simulink model "TwoNeuronTest"  (R2016b)
settings: Solver=VariableStepAuto  StartTime=0.0  StopTime=15  RelTol=1e-3  EnableMultiTasking=on
libraries: simulink x2, powerlib_meascontrol x1
settings Model: Creator=ramin  LastModifiedBy=ramin
settings DataIOCC: LimitDataPoints=on
settings OptimizationCC: LifeSpan=inf
settings DebuggingCC: AllowSymbolicDim=off  SFUnexpectedBacktrackingDiag=warning  SFNoUnconditionalDefaultTransitionDiag=warning  SFExecutionAtInitializationDiag=none
settings ModelReferenceCC: PropagateSignalLabelsOutOfModel=off
settings GRTTargetCC: TargetLangStandard=C89/C90 (ANSI)
settings ConfigComp: CovMetricSettings=dw  CovHtmlReporting=on  CovSaveCumulativeToWorkspaceVar=on  CovSaveSingleToWorkspaceVar=on  CovExternalEMLEnable=off

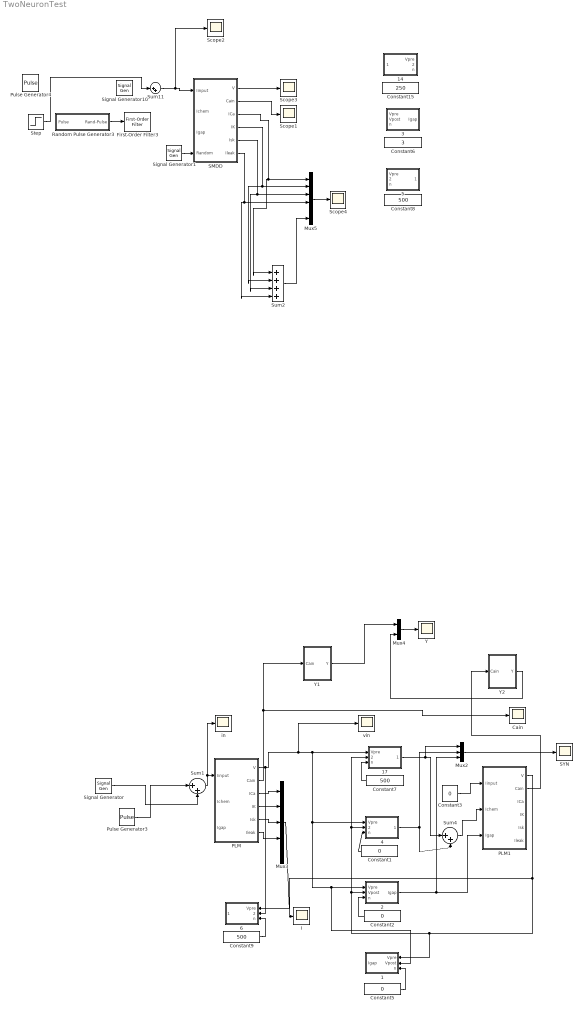
== system TwoNeuronTest ==
  1 : Subsystem
  14 : Subsystem
  17 : Subsystem
  2 : Subsystem
  3 : Subsystem
  4 : Subsystem
  5 : Subsystem
  6 : Subsystem
  Cain : Scope
  Constant{1..3,5} (4 alike) : Constant  Value=0
  Constant15 : Constant  Value=250
  Constant6 : Constant  Value=3
  Constant7 : Constant  Value=500
  Constant8 : Constant  Value=500
  Constant9 : Constant  Value=500
  First-Order Filter3 : powerlib_meascontrol/Filters/First-Order Filter  FilterType=Lowpass  Tc=1  Ts=0  Initialize=off  Vac_Init=[0, 0, 60]  Vdc_Init=0  PlotResponse=off  FreqRange="[0,  200,  1]"
  I : Scope
  Mux2 : Mux  Inputs=3
  Mux3 : Mux  Inputs=5
  Mux4 : Mux  Inputs=2
  Mux5 : Mux  Inputs=6
  PLM : Subsystem
  PLM1 : Subsystem
  Pulse Generator3 : DiscretePulseGenerator  PulseType=Time based  Amplitude=2500  Period=20  PulseWidth=50  PhaseDelay=2
  Pulse Generator4 : DiscretePulseGenerator  PulseType=Time based  Amplitude=2000  Period=200  PulseWidth=80  PhaseDelay=2
  Random Pulse Generator3 : Subsystem
  SMDD : Subsystem
  SYN : Scope
  Scope{1..4} (4 alike) : Scope
  Signal Generator : SignalGenerator  WaveForm=random  Amplitude=0  Frequency=1000000
  Signal Generator1 : SignalGenerator  WaveForm=random  Amplitude=0.5
  Signal Generator10 : SignalGenerator  WaveForm=random  Amplitude=0  Frequency=100
  Step : Step  Time=50  After=2000  SampleTime=0
  Sum1 : Sum  Inputs=|++
  Sum11 : Sum  Inputs=|++
  Sum2 : Sum  Inputs=|++++
  Sum4 : Sum  Inputs=|++
  Y : Scope
  Y1 : Subsystem
  Y2 : Subsystem
  in : Scope
  vin : Scope
  wires:
  PLM/2("Cain ") -> Cain/1, Y1/1(Cain)
  Sum4/1 -> PLM1/2(Ichem)
  Constant1/1 -> 4/3(n)
  Constant7/1 -> 17/3(n)
  Constant2/1 -> 2/3(n)
  4/1(Ichem) -> Sum4/2, Mux2/2
  PLM1/1(V) -> 6/1(Vpre), 1/1(Vpre), 17/2(Vpost), 4/2(Vpost), 2/2(Vpost)
  17/1(Ichem) -> Mux2/1, Sum4/1
  Constant3/1 -> PLM1/1(Iinput)
  PLM1/2("Cain ") -> Y2/1(Cain)
  PLM/1(V) -> vin/1, 17/1(Vpre), 4/1(Vpre), 1/2(Vpost), 2/1(Vpre), 6/2(Vpost)
  2/1(Igap) -> PLM1/3(Igap), Mux2/3
  Mux2/1 -> SYN/1
  Mux3/1 -> I/1
  PLM/3(ICa) -> Mux3/1
  PLM/4(IK) -> Mux3/2
  PLM/5(Isk) -> Mux3/3
  PLM/6(Ileak) -> Mux3/4
  Constant5/1 -> 1/3(n)
  Sum1/1 -> in/1, PLM/1(Iinput)
  Pulse Generator3/1 -> Sum1/1
  Signal Generator/1 -> Sum1/2
  Y1/1(Y) -> Mux4/1
  Mux4/1 -> Y/1
  Y2/1(Y) -> Mux4/2
  Signal Generator1/1 -> SMDD/4(Random)
  Random Pulse Generator3/1(Rand-Pulse) -> First-Order Filter3/1
  Sum11/1 -> Scope2/1, SMDD/1(Iinput)
  Step/1 -> Sum11/1
  SMDD/1(V) -> Scope3/1
  SMDD/2("Cain ") -> Scope1/1
  SMDD/3(ICa) -> Sum2/1, Mux5/1
  SMDD/4(IK) -> Sum2/2, Mux5/2
  SMDD/5(Isk) -> Sum2/3, Mux5/3
  SMDD/6(Ileak) -> Sum2/4, Mux5/4
  Sum2/1 -> Mux5/6
  Mux5/1 -> Scope4/1
  Constant9/1 -> 6/3(n)

== system TwoNeuronTest/1 ==
  Vpre : Inport
  Vpost : Inport  Port=2
  n : Inport  Port=3
  Ggap : Constant  Value=1.02
  Product2 : Product  Inputs=3
  Sum6 : Sum  Inputs=|+-
  Igap : Outport
  wires:
  Vpre/1 -> Sum6/1
  n/1 -> Product2/2
  Sum6/1 -> Product2/1
  Product2/1 -> Igap/1  "Igap"
  Vpost/1 -> Sum6/2
  Ggap/1 -> Product2/3

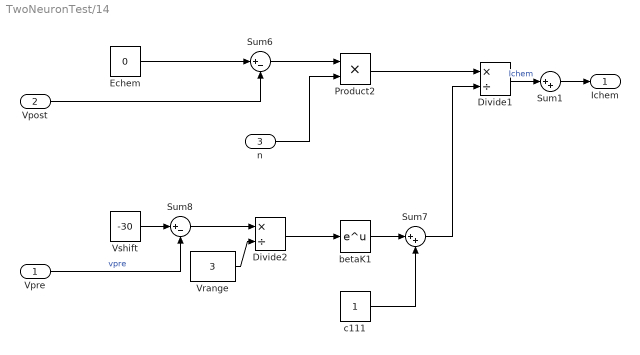
== system TwoNeuronTest/14 ==
  Vpre : Inport
  Vpost : Inport  Port=2
  n : Inport  Port=3
  Divide1 : Product  Inputs=*/
  Divide2 : Product  Inputs=*/
  Echem : Constant  Value=0
  Product2 : Product
  Sum1 : Sum  Inputs=|++
  Sum6 : Sum  Inputs=|+-
  Sum7 : Sum  Inputs=|++
  Sum8 : Sum  Inputs=|+-
  Vrange : Constant  Value=3
  Vshift : Constant  Value=-30
  betaK1 : Math  SaturateOnIntegerOverflow=on
  c111 : Constant
  Ichem : Outport
  wires:
  Echem/1 -> Sum6/1
  n/1 -> Product2/2
  Sum6/1 -> Product2/1
  Product2/1 -> Divide1/1
  betaK1/1 -> Sum7/1
  c111/1 -> Sum7/2
  Vshift/1 -> Sum8/1
  Vpre/1 -> Sum8/2  "vpre"
  Sum8/1 -> Divide2/1
  Vrange/1 -> Divide2/2
  Divide2/1 -> betaK1/1
  Sum7/1 -> Divide1/2
  Divide1/1 -> Sum1/1  "Ichem"
  Vpost/1 -> Sum6/2
  Sum1/1 -> Ichem/1

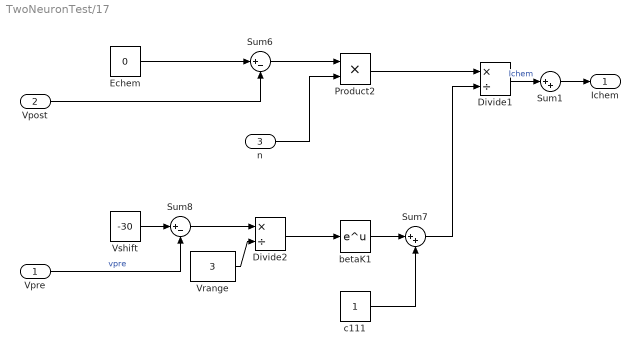
== system TwoNeuronTest/17 ==
  Vpre : Inport
  Vpost : Inport  Port=2
  n : Inport  Port=3
  Divide1 : Product  Inputs=*/
  Divide2 : Product  Inputs=*/
  Echem : Constant  Value=0
  Product2 : Product
  Sum1 : Sum  Inputs=|++
  Sum6 : Sum  Inputs=|+-
  Sum7 : Sum  Inputs=|++
  Sum8 : Sum  Inputs=|+-
  Vrange : Constant  Value=3
  Vshift : Constant  Value=-30
  betaK1 : Math  SaturateOnIntegerOverflow=on
  c111 : Constant
  Ichem : Outport
  wires:
  Echem/1 -> Sum6/1
  n/1 -> Product2/2
  Sum6/1 -> Product2/1
  Product2/1 -> Divide1/1
  betaK1/1 -> Sum7/1
  c111/1 -> Sum7/2
  Vshift/1 -> Sum8/1
  Vpre/1 -> Sum8/2  "vpre"
  Sum8/1 -> Divide2/1
  Vrange/1 -> Divide2/2
  Divide2/1 -> betaK1/1
  Sum7/1 -> Divide1/2
  Divide1/1 -> Sum1/1  "Ichem"
  Vpost/1 -> Sum6/2
  Sum1/1 -> Ichem/1

== system TwoNeuronTest/2 ==
  Vpre : Inport
  Vpost : Inport  Port=2
  n : Inport  Port=3
  Ggap : Constant  Value=1.02
  Product2 : Product  Inputs=3
  Sum6 : Sum  Inputs=|+-
  Igap : Outport
  wires:
  Vpre/1 -> Sum6/1
  n/1 -> Product2/2
  Sum6/1 -> Product2/1
  Product2/1 -> Igap/1  "Igap"
  Vpost/1 -> Sum6/2
  Ggap/1 -> Product2/3

== system TwoNeuronTest/3 ==
  Vpre : Inport
  Vpost : Inport  Port=2
  n : Inport  Port=3
  Ggap : Constant  Value=10
  Product2 : Product  Inputs=3
  Sum6 : Sum  Inputs=|+-
  Igap : Outport
  wires:
  Vpre/1 -> Sum6/1
  n/1 -> Product2/2
  Sum6/1 -> Product2/1
  Product2/1 -> Igap/1  "Igap"
  Vpost/1 -> Sum6/2
  Ggap/1 -> Product2/3

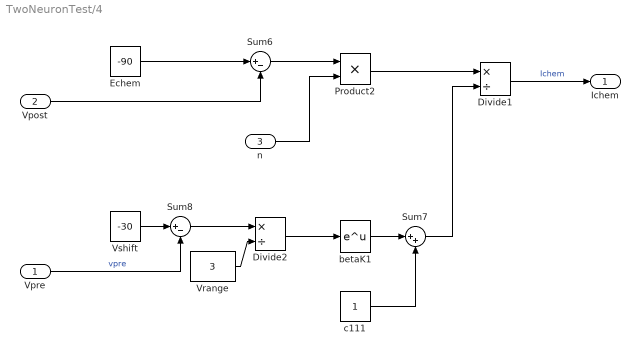
== system TwoNeuronTest/4 ==
  Vpre : Inport
  Vpost : Inport  Port=2
  n : Inport  Port=3
  Divide1 : Product  Inputs=*/
  Divide2 : Product  Inputs=*/
  Echem : Constant  Value=-90
  Product2 : Product
  Sum6 : Sum  Inputs=|+-
  Sum7 : Sum  Inputs=|++
  Sum8 : Sum  Inputs=|+-
  Vrange : Constant  Value=3
  Vshift : Constant  Value=-30
  betaK1 : Math  SaturateOnIntegerOverflow=on
  c111 : Constant
  Ichem : Outport
  wires:
  Echem/1 -> Sum6/1
  n/1 -> Product2/2
  Sum6/1 -> Product2/1
  Product2/1 -> Divide1/1
  betaK1/1 -> Sum7/1
  c111/1 -> Sum7/2
  Vshift/1 -> Sum8/1
  Vpre/1 -> Sum8/2  "vpre"
  Sum8/1 -> Divide2/1
  Vrange/1 -> Divide2/2
  Divide2/1 -> betaK1/1
  Sum7/1 -> Divide1/2
  Divide1/1 -> Ichem/1  "Ichem"
  Vpost/1 -> Sum6/2

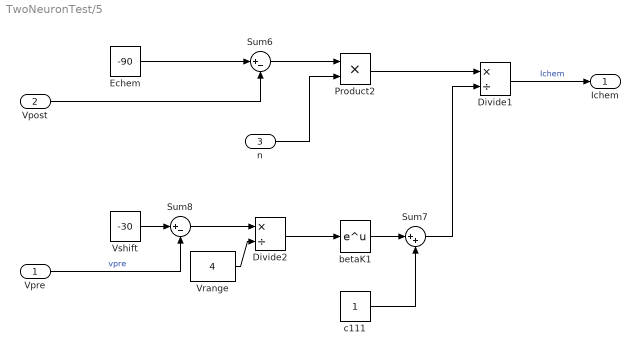
== system TwoNeuronTest/5 ==
  Vpre : Inport
  Vpost : Inport  Port=2
  n : Inport  Port=3
  Divide1 : Product  Inputs=*/
  Divide2 : Product  Inputs=*/
  Echem : Constant  Value=-90
  Product2 : Product
  Sum6 : Sum  Inputs=|+-
  Sum7 : Sum  Inputs=|++
  Sum8 : Sum  Inputs=|+-
  Vrange : Constant  Value=4
  Vshift : Constant  Value=-30
  betaK1 : Math  SaturateOnIntegerOverflow=on
  c111 : Constant
  Ichem : Outport
  wires:
  Echem/1 -> Sum6/1
  n/1 -> Product2/2
  Sum6/1 -> Product2/1
  Product2/1 -> Divide1/1
  betaK1/1 -> Sum7/1
  c111/1 -> Sum7/2
  Vshift/1 -> Sum8/1
  Vpre/1 -> Sum8/2  "vpre"
  Sum8/1 -> Divide2/1
  Vrange/1 -> Divide2/2
  Divide2/1 -> betaK1/1
  Sum7/1 -> Divide1/2
  Divide1/1 -> Ichem/1  "Ichem"
  Vpost/1 -> Sum6/2

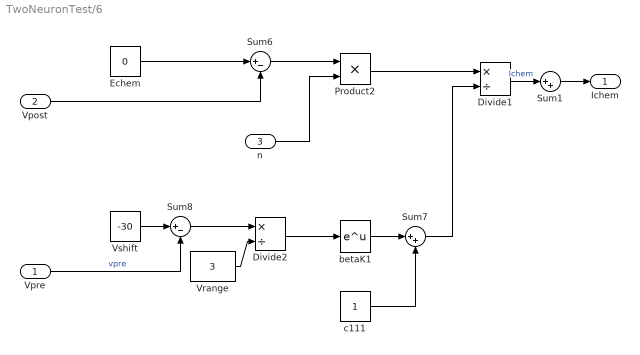
== system TwoNeuronTest/6 ==
  Vpre : Inport
  Vpost : Inport  Port=2
  n : Inport  Port=3
  Divide1 : Product  Inputs=*/
  Divide2 : Product  Inputs=*/
  Echem : Constant  Value=0
  Product2 : Product
  Sum1 : Sum  Inputs=|++
  Sum6 : Sum  Inputs=|+-
  Sum7 : Sum  Inputs=|++
  Sum8 : Sum  Inputs=|+-
  Vrange : Constant  Value=3
  Vshift : Constant  Value=-30
  betaK1 : Math  SaturateOnIntegerOverflow=on
  c111 : Constant
  Ichem : Outport
  wires:
  Echem/1 -> Sum6/1
  n/1 -> Product2/2
  Sum6/1 -> Product2/1
  Product2/1 -> Divide1/1
  betaK1/1 -> Sum7/1
  c111/1 -> Sum7/2
  Vshift/1 -> Sum8/1
  Vpre/1 -> Sum8/2  "vpre"
  Sum8/1 -> Divide2/1
  Vrange/1 -> Divide2/2
  Divide2/1 -> betaK1/1
  Sum7/1 -> Divide1/2
  Divide1/1 -> Sum1/1  "Ichem"
  Vpost/1 -> Sum6/2
  Sum1/1 -> Ichem/1

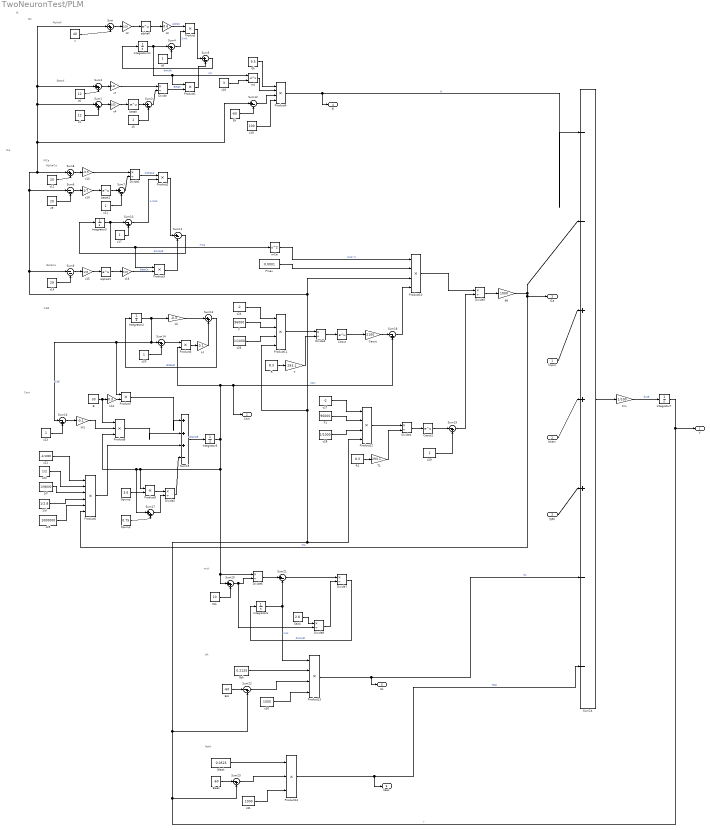
== system TwoNeuronTest/PLM ==
  note: Isk
  note: msk
  note: ICa
  note: Cain
  note: CaB
  note: BetaCa
  note: AlphaCa
  note: MCa
  note: IK
  note: Mk
  note: BetaK
  note: AlphaK
  note: Ileak
  Iinput : Inport
  Ichem : Inport  Port=2
  Igap : Inport  Port=3
  1/F : Constant  Value=1/96000
  1/d : Constant  Value=1/2.8
  B : Constant  Value=30
  Caout : Math  SaturateOnIntegerOverflow=on
  "Caout " : Gain  Gain=2100
  Caout1 : Math  SaturateOnIntegerOverflow=on
  "Cm " : Gain  Gain=1/100
  Divide{,1..8} (9 alike) : Product  Inputs=*/
  "Ek " : Constant  Value=-60
  Eleak : Constant  Value=-60
  Esk : Constant  Value=-60
  F : Constant  Value=96000
  F1 : Constant  Value=96000
  "Gk " : Constant  Value=9.5
  Gleak : Constant  Value=0.0525
  Gpump : Constant  Value=3.6
  Gsk : Constant  Value=0.2125
  Integrator3 : Integrator  InitialCondition=0.001
  Integrator4 : Integrator
  Integrator5 : Integrator
  Integrator6 : Integrator  InitialCondition=1
  Integrator7 : Integrator  InitialCondition=-60
  Integratormk : Integrator
  Kpump : Constant  Value=0.75
  Ksk : Constant  Value=10
  Pmax : Constant  Value=0.0001
  Product{,1..3,5,7,9} (7 alike) : Product
  Product{4,10..13} (5 alike) : Product  Inputs=4
  Product14 : Product  Inputs=3
  Product6 : Product  Inputs=6
  Product8 : Product  Inputs=3
  R : Constant  Value=8.3
  R1 : Constant  Value=8.3
  Saisk : Constant  Value=2.8
  Sum{,1,3,8,13,17,20} (7 alike) : Sum  Inputs=|++
  Sum{4,10,14,16,18..19,22..23} (8 alike) : Sum  Inputs=|-+
  Sum{2,5,7,11..12,21} (6 alike) : Sum  Inputs=|+-
  Sum15 : Sum  Inputs=|+++-
  Sum24 : Sum  Inputs=|--+++--
  Sum6 : Sum  Inputs=|--
  Sum9 : Sum  Inputs=|--
  T : Gain  Gain=293.1
  T1 : Gain  Gain=293.1
  alphaK : Math  SaturateOnIntegerOverflow=on
  alphaK1 : Math  SaturateOnIntegerOverflow=on
  betaK : Math  SaturateOnIntegerOverflow=on
  betaK1 : Math  SaturateOnIntegerOverflow=on
  c : Constant  Value=40
  c1 : Constant  Value=12
  c10 : Gain  Gain=1/7
  c{5,8,11,17,20,23,29} (7 alike) : Constant
  c12 : Constant  Value=20
  c13 : Gain  Gain=-0.5
  c14 : Constant  Value=29
  c15 : Gain  Gain=1/10
  c16 : Gain  Gain=0.23
  c18 : Constant  Value=3
  c19 : Constant  Value=100
  c2 : Gain  Gain=1/20
  c21 : Constant  Value=-1/1000
  c22 : Constant  Value=1/2
  c24 : Constant  Value=-2
  c25 : Constant  Value=1000000
  c26 : Constant  Value=1/1000
  c27 : Constant  Value=-2
  c28 : Constant  Value=1/1000
  c3 : Gain  Gain=0.6
  c30 : Constant  Value=1000
  c31 : Constant  Value=1000
  c4 : Gain  Gain=1/23
  c6 : Constant  Value=12
  c7 : Gain  Gain=0.01
  c9 : Constant  Value=20
  "gg " : Gain  Gain=1000
  kb : Gain  Gain=-0.3
  kb1 : Gain  Gain=0.3
  kf : Gain  Gain=0.1
  kf1 : Gain  Gain=-0.1
  mCa : Math  Operator=square  SaturateOnIntegerOverflow=on
  mk : Math  Operator=pow  SaturateOnIntegerOverflow=on
  V : Outport
  "Cain " : Outport  Port=2
  ICa : Outport  Port=3
  IK : Outport  Port=4
  Isk : Outport  Port=5
  Ileak : Outport  Port=6
  wires:
  Divide/1 -> Product1/2  "BetaK"
  c10/1 -> betaK1/1
  Sum7/1 -> Divide1/2
  c/1 -> Sum/2
  R/1 -> T/1
  c3/1 -> Product/1  "alphaK"
  c9/1 -> Sum6/2
  c6/1 -> Sum3/2
  Product/1 -> Sum5/1
  Sum1/1 -> c4/1
  c13/1 -> Divide1/1
  Caout1/1 -> Sum19/1
  Eleak/1 -> Sum23/1
  T/1 -> Divide3/2
  Ksk/1 -> Sum20/2
  Product14/1 -> Ileak/1, Sum24/7  "Ileak"
  Sum24/1 -> "Cm "/1
  Esk/1 -> Sum22/1
  "Cm "/1 -> Integrator7/1  "dv/dt"
  Divide3/1 -> Caout/1
  c31/1 -> Product14/3
  Integrator6/1 -> Sum21/2, Product13/1  "msk"
  Sum21/1 -> Divide7/1
  Sum23/1 -> Product14/2
  Divide6/1 -> Sum21/1
  c12/1 -> Sum8/2
  Integrator3/1 -> Product3/1, mCa/1, Sum10/1  "mCa"
  Sum5/1 -> Integratormk/1  "dmk/dt"
  c15/1 -> alphaK1/1
  Sum9/1 -> c15/1
  c2/1 -> alphaK/1
  Sum22/1 -> Product13/3
  Product10/1 -> Divide5/1
  Integratormk/1 -> mk/1, Product1/1, Sum4/1  "mk"
  Divide8/1 -> Divide7/2
  R1/1 -> T1/1
  Caout/1 -> "Caout "/1
  Sum3/1 -> c7/1
  Sum6/1 -> c10/1
  Divide4/1 -> Caout1/1
  c30/1 -> Product13/4
  Gleak/1 -> Product14/1
  c28/1 -> Product12/3
  c11/1 -> Sum7/2
  betaK1/1 -> Sum7/1
  Divide7/1 -> Integrator6/1  "dmsk/dt"
  Ichem/1 -> Sum24/4
  c7/1 -> Divide/1
  Sum14/1 -> Product5/1
  Sum13/1 -> Integrator4/1  "dCaB/dt"
  Integrator5/1 -> Sum20/1, Divide6/1, Product9/1, Sum17/1, Product8/3, "Cain "/1, Sum18/2, Product5/2  "Cain"
  c21/1 -> Product6/1
  c22/1 -> Product6/2
  1/F/1 -> Product6/3
  1/d/1 -> Product6/4
  c25/1 -> Product6/5
  "gg "/1 -> Sum24/2, ICa/1, Product6/6  "ICa"
  B/1 -> Product8/1, kb1/1
  kb1/1 -> Product7/2
  Product7/1 -> Sum15/1
  Product5/1 -> kf/1
  kf/1 -> Sum13/2
  c23/1 -> Sum16/2
  Sum16/1 -> kf1/1
  kf1/1 -> Product8/2
  Product8/1 -> Sum15/2
  Product6/1 -> Sum15/3
  Gpump/1 -> Product9/2
  Product9/1 -> Divide2/1
  Kpump/1 -> Sum17/2
  Sum17/1 -> Divide2/2
  Divide2/1 -> Sum15/4
  Sum15/1 -> Integrator5/1  "dCain/dt"
  mCa/1 -> Product10/1  "mCa^2"
  Pmax/1 -> Product10/2
  c24/1 -> Product11/1
  F/1 -> Product11/2
  c26/1 -> Product11/3
  Integrator7/1 -> V/1, Sum22/2, Product11/4, Product10/3, Sum6/1, Sum1/1, Sum3/1, Sum/1, Sum12/1, Sum8/1, Sum9/1, Product12/4, Sum23/2  "v"
  c14/1 -> Sum9/2
  Saisk/1 -> Divide8/1
  Sum18/1 -> Product10/4
  Iinput/1 -> Sum24/3
  "Caout "/1 -> Sum18/1
  Sum/1 -> c2/1
  Sum8/1 -> c13/1
  c16/1 -> Product3/2  "BetaCa"
  Product11/1 -> Divide3/1
  T1/1 -> Divide4/2
  betaK/1 -> Sum2/1
  c29/1 -> Sum19/2
  Product1/1 -> Sum5/2
  c4/1 -> betaK/1
  alphaK/1 -> c3/1
  alphaK1/1 -> c16/1
  Divide1/1 -> Product2/1  "AlphaCa"
  Sum2/1 -> Divide/2
  Sum4/1 -> Product/2  "1-mk"
  c5/1 -> Sum2/2
  c8/1 -> Sum4/2
  Igap/1 -> Sum24/5
  Product13/1 -> Isk/1, Sum24/6  "Isk"
  Divide5/1 -> "gg "/1
  Sum20/1 -> Divide8/2, Divide6/2
  Gsk/1 -> Product13/2
  Product12/1 -> Divide4/1
  c27/1 -> Product12/1
  F1/1 -> Product12/2
  c1/1 -> Sum1/2
  Sum11/1 -> Integrator3/1  "dmCa/dt"
  c17/1 -> Sum10/2
  "Ek "/1 -> Sum12/2
  Sum10/1 -> Product2/2  "1-mCa"
  Sum12/1 -> Product4/3
  Product3/1 -> Sum11/2
  Product4/1 -> IK/1, Sum24/1  "IK"
  Integrator4/1 -> Product7/1, Sum16/1, Sum14/1, kb/1  "CaB"
  kb/1 -> Sum13/1
  c20/1 -> Sum14/2
  mk/1 -> Product4/2
  "Gk "/1 -> Product4/1
  c19/1 -> Product4/4
  Product2/1 -> Sum11/1
  c18/1 -> mk/2
  Sum19/1 -> Divide5/2

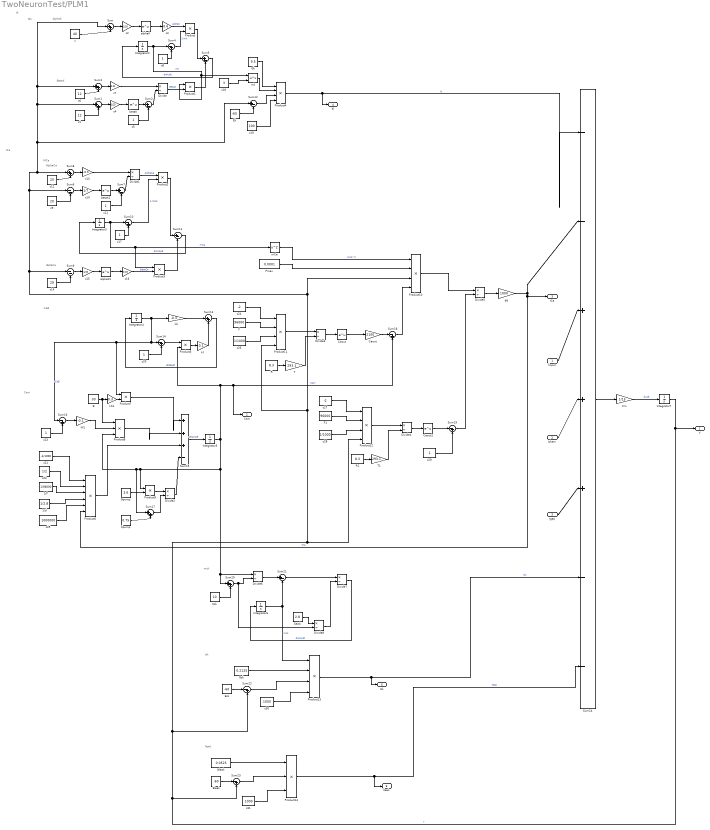
== system TwoNeuronTest/PLM1 ==
  note: Isk
  note: msk
  note: ICa
  note: Cain
  note: CaB
  note: BetaCa
  note: AlphaCa
  note: MCa
  note: IK
  note: Mk
  note: BetaK
  note: AlphaK
  note: Ileak
  Iinput : Inport
  Ichem : Inport  Port=2
  Igap : Inport  Port=3
  1/F : Constant  Value=1/96000
  1/d : Constant  Value=1/2.8
  B : Constant  Value=30
  Caout : Math  SaturateOnIntegerOverflow=on
  "Caout " : Gain  Gain=2100
  Caout1 : Math  SaturateOnIntegerOverflow=on
  "Cm " : Gain  Gain=1/15
  Divide{,1..8} (9 alike) : Product  Inputs=*/
  "Ek " : Constant  Value=-60
  Eleak : Constant  Value=-60
  Esk : Constant  Value=-60
  F : Constant  Value=96000
  F1 : Constant  Value=96000
  "Gk " : Constant  Value=9.5
  Gleak : Constant  Value=0.0525
  Gpump : Constant  Value=3.6
  Gsk : Constant  Value=0.2125
  Integrator2 : Integrator
  Integrator3 : Integrator  InitialCondition=0.001
  Integrator4 : Integrator
  Integrator5 : Integrator
  Integrator6 : Integrator  InitialCondition=1
  Integrator7 : Integrator  InitialCondition=-60
  Kpump : Constant  Value=0.75
  Ksk : Constant  Value=10
  Pmax : Constant  Value=0.0001
  Product{,1..3,5,7,9} (7 alike) : Product
  Product{4,10..13} (5 alike) : Product  Inputs=4
  Product14 : Product  Inputs=3
  Product6 : Product  Inputs=6
  Product8 : Product  Inputs=3
  R : Constant  Value=8.3
  R1 : Constant  Value=8.3
  Saisk : Constant  Value=2.8
  Sum{,1,3,8,13,17,20} (7 alike) : Sum  Inputs=|++
  Sum{4,10,14,16,18..19,22..23} (8 alike) : Sum  Inputs=|-+
  Sum{2,5,7,11..12,21} (6 alike) : Sum  Inputs=|+-
  Sum15 : Sum  Inputs=|+++-
  Sum24 : Sum  Inputs=|--+++--
  Sum6 : Sum  Inputs=|--
  Sum9 : Sum  Inputs=|--
  T : Gain  Gain=293.1
  T1 : Gain  Gain=293.1
  alphaK : Math  SaturateOnIntegerOverflow=on
  alphaK1 : Math  SaturateOnIntegerOverflow=on
  betaK : Math  SaturateOnIntegerOverflow=on
  betaK1 : Math  SaturateOnIntegerOverflow=on
  c : Constant  Value=40
  c1 : Constant  Value=12
  c10 : Gain  Gain=1/7
  c{5,8,11,17,20,23,29} (7 alike) : Constant
  c12 : Constant  Value=20
  c13 : Gain  Gain=-0.5
  c14 : Constant  Value=29
  c15 : Gain  Gain=1/10
  c16 : Gain  Gain=0.23
  c18 : Constant  Value=3
  c19 : Constant  Value=100
  c2 : Gain  Gain=1/20
  c21 : Constant  Value=-1/1000
  c22 : Constant  Value=1/2
  c24 : Constant  Value=-2
  c25 : Constant  Value=1000000
  c26 : Constant  Value=1/1000
  c27 : Constant  Value=-2
  c28 : Constant  Value=1/1000
  c3 : Gain  Gain=0.6
  c30 : Constant  Value=1000
  c31 : Constant  Value=1000
  c4 : Gain  Gain=1/23
  c6 : Constant  Value=12
  c7 : Gain  Gain=0.01
  c9 : Constant  Value=20
  "gg " : Gain  Gain=1000
  kb : Gain  Gain=-0.3
  kb1 : Gain  Gain=0.3
  kf : Gain  Gain=0.1
  kf1 : Gain  Gain=-0.1
  mCa : Math  Operator=square  SaturateOnIntegerOverflow=on
  mk : Math  Operator=pow  SaturateOnIntegerOverflow=on
  V : Outport
  "Cain " : Outport  Port=2
  ICa : Outport  Port=3
  IK : Outport  Port=4
  Isk : Outport  Port=5
  Ileak : Outport  Port=6
  wires:
  Divide/1 -> Product1/2  "BetaK"
  c10/1 -> betaK1/1
  Sum7/1 -> Divide1/2
  c/1 -> Sum/2
  R/1 -> T/1
  c3/1 -> Product/1  "alphaK"
  c9/1 -> Sum6/2
  c6/1 -> Sum3/2
  Product/1 -> Sum5/1
  Sum1/1 -> c4/1
  c13/1 -> Divide1/1
  Caout1/1 -> Sum19/1
  Eleak/1 -> Sum23/1
  T/1 -> Divide3/2
  Ksk/1 -> Sum20/2
  Product14/1 -> Ileak/1, Sum24/7  "Ileak"
  Sum24/1 -> "Cm "/1
  Esk/1 -> Sum22/1
  "Cm "/1 -> Integrator7/1  "dv/dt"
  Divide3/1 -> Caout/1
  c31/1 -> Product14/3
  Integrator6/1 -> Sum21/2, Product13/1  "msk"
  Sum21/1 -> Divide7/1
  Sum23/1 -> Product14/2
  Divide6/1 -> Sum21/1
  c12/1 -> Sum8/2
  Integrator3/1 -> Product3/1, mCa/1, Sum10/1  "mCa"
  Sum5/1 -> Integrator2/1  "dmk/dt"
  c15/1 -> alphaK1/1
  Sum9/1 -> c15/1
  c2/1 -> alphaK/1
  Sum22/1 -> Product13/3
  Product10/1 -> Divide5/1
  Integrator2/1 -> mk/1, Product1/1, Sum4/1  "mk"
  Divide8/1 -> Divide7/2
  R1/1 -> T1/1
  Caout/1 -> "Caout "/1
  Sum3/1 -> c7/1
  Sum6/1 -> c10/1
  Divide4/1 -> Caout1/1
  c30/1 -> Product13/4
  Gleak/1 -> Product14/1
  c28/1 -> Product12/3
  c11/1 -> Sum7/2
  betaK1/1 -> Sum7/1
  Divide7/1 -> Integrator6/1  "dmsk/dt"
  Ichem/1 -> Sum24/4
  c7/1 -> Divide/1
  Sum14/1 -> Product5/1
  Sum13/1 -> Integrator4/1  "dCaB/dt"
  Integrator5/1 -> Sum20/1, Divide6/1, Product9/1, Sum17/1, Product8/3, "Cain "/1, Sum18/2, Product5/2  "Cain"
  c21/1 -> Product6/1
  c22/1 -> Product6/2
  1/F/1 -> Product6/3
  1/d/1 -> Product6/4
  c25/1 -> Product6/5
  "gg "/1 -> Sum24/2, ICa/1, Product6/6  "ICa"
  B/1 -> Product8/1, kb1/1
  kb1/1 -> Product7/2
  Product7/1 -> Sum15/1
  Product5/1 -> kf/1
  kf/1 -> Sum13/2
  c23/1 -> Sum16/2
  Sum16/1 -> kf1/1
  kf1/1 -> Product8/2
  Product8/1 -> Sum15/2
  Product6/1 -> Sum15/3
  Gpump/1 -> Product9/2
  Product9/1 -> Divide2/1
  Kpump/1 -> Sum17/2
  Sum17/1 -> Divide2/2
  Divide2/1 -> Sum15/4
  Sum15/1 -> Integrator5/1  "dCain/dt"
  mCa/1 -> Product10/1  "mCa^2"
  Pmax/1 -> Product10/2
  c24/1 -> Product11/1
  F/1 -> Product11/2
  c26/1 -> Product11/3
  Integrator7/1 -> V/1, Sum22/2, Product11/4, Product10/3, Sum6/1, Sum1/1, Sum3/1, Sum/1, Sum12/1, Sum8/1, Sum9/1, Product12/4, Sum23/2  "v"
  c14/1 -> Sum9/2
  Saisk/1 -> Divide8/1
  Sum18/1 -> Product10/4
  Iinput/1 -> Sum24/3
  "Caout "/1 -> Sum18/1
  Sum/1 -> c2/1
  Sum8/1 -> c13/1
  c16/1 -> Product3/2  "BetaCa"
  Product11/1 -> Divide3/1
  T1/1 -> Divide4/2
  betaK/1 -> Sum2/1
  c29/1 -> Sum19/2
  Product1/1 -> Sum5/2
  c4/1 -> betaK/1
  alphaK/1 -> c3/1
  alphaK1/1 -> c16/1
  Divide1/1 -> Product2/1  "AlphaCa"
  Sum2/1 -> Divide/2
  Sum4/1 -> Product/2  "1-mk"
  c5/1 -> Sum2/2
  c8/1 -> Sum4/2
  Igap/1 -> Sum24/5
  Product13/1 -> Isk/1, Sum24/6  "Isk"
  Divide5/1 -> "gg "/1
  Sum20/1 -> Divide8/2, Divide6/2
  Gsk/1 -> Product13/2
  Product12/1 -> Divide4/1
  c27/1 -> Product12/1
  F1/1 -> Product12/2
  c1/1 -> Sum1/2
  Sum11/1 -> Integrator3/1  "dmCa/dt"
  c17/1 -> Sum10/2
  "Ek "/1 -> Sum12/2
  Sum10/1 -> Product2/2  "1-mCa"
  Sum12/1 -> Product4/3
  Product3/1 -> Sum11/2
  Product4/1 -> IK/1, Sum24/1  "IK"
  Integrator4/1 -> Product7/1, Sum16/1, Sum14/1, kb/1  "CaB"
  kb/1 -> Sum13/1
  c20/1 -> Sum14/2
  mk/1 -> Product4/2
  "Gk "/1 -> Product4/1
  c19/1 -> Product4/4
  Product2/1 -> Sum11/1
  c18/1 -> mk/2
  Sum19/1 -> Divide5/2

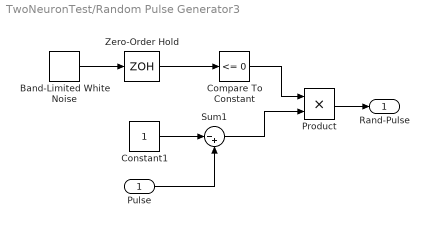
== system TwoNeuronTest/Random Pulse Generator3 ==
  Pulse : Inport
  Band-Limited White Noise : simulink/Sources/Band-Limited White Noise  Cov=1  Ts=10  seed=22
  Compare To Constant : simulink/Logic and Bit Operations/Compare To Constant  relop=<=  const=0  OutDataTypeStr=boolean
  Constant1 : Constant
  Product : Product
  Sum1 : Sum  Inputs=|-+
  Zero-Order Hold : ZeroOrderHold  SampleTime=-1
  Rand-Pulse : Outport
  wires:
  Constant1/1 -> Sum1/1
  Sum1/1 -> Product/2
  Zero-Order Hold/1 -> Compare To Constant/1
  Product/1 -> Rand-Pulse/1
  Pulse/1 -> Sum1/2
  Band-Limited White Noise/1 -> Zero-Order Hold/1
  Compare To Constant/1 -> Product/1

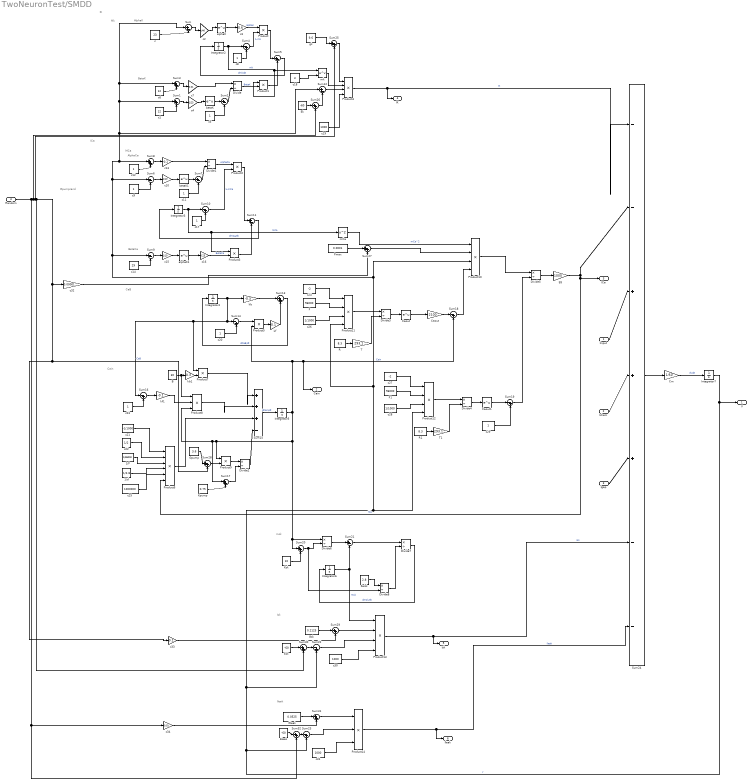
== system TwoNeuronTest/SMDD ==
  note: Gpumprand
  note: Isk
  note: msk
  note: ICa
  note: Cain
  note: CaB
  note: BetaCa
  note: AlphaCa
  note: MCa
  note: IK
  note: Mk
  note: BetaK
  note: AlphaK
  note: Ileak
  Iinput : Inport
  Ichem : Inport  Port=2
  Igap : Inport  Port=3
  Random : Inport  Port=4
  1/F : Constant  Value=1/96000
  1/d : Constant  Value=1/2.8
  B : Constant  Value=30
  Caout : Math  SaturateOnIntegerOverflow=on
  "Caout " : Gain  Gain=2100
  Caout1 : Math  SaturateOnIntegerOverflow=on
  "Cm " : Gain  Gain=1/50
  Divide{,1..8} (9 alike) : Product  Inputs=*/
  "Ek " : Constant  Value=-60
  Eleak : Constant  Value=-60
  Esk : Constant  Value=-60
  F : Constant  Value=96000
  F1 : Constant  Value=96000
  Gleak : Constant  Value=0.0525
  Gpump : Constant  Value=3.6
  Gsk : Constant  Value=0.2125
  Integrator2 : Integrator
  Integrator3 : Integrator  InitialCondition=0.001
  Integrator4 : Integrator
  Integrator5 : Integrator
  Integrator6 : Integrator  InitialCondition=1
  Integrator7 : Integrator  InitialCondition=-60
  Kpump : Constant  Value=0.75
  Ksk : Constant  Value=10
  Pmax : Constant  Value=0.0001
  Product{,1..3,5,7,9} (7 alike) : Product
  Product{4,10..13} (5 alike) : Product  Inputs=4
  Product14 : Product  Inputs=3
  Product6 : Product  Inputs=6
  Product8 : Product  Inputs=3
  R : Constant  Value=8.3
  R1 : Constant  Value=8.3
  Saisk : Constant  Value=2.8
  Sum{,2,5,7,11..12,21} (7 alike) : Sum  Inputs=|+-
  Sum{1,3,8,13,17,20,25..32} (14 alike) : Sum  Inputs=|++
  Sum{4,10,14,16,18..19,22..23} (8 alike) : Sum  Inputs=|-+
  Sum15 : Sum  Inputs=|+++-
  Sum24 : Sum  Inputs=|--+++--
  Sum6 : Sum  Inputs=|--
  Sum9 : Sum  Inputs=|--
  T : Gain  Gain=293.1
  T1 : Gain  Gain=293.1
  alphaK : Math  SaturateOnIntegerOverflow=on
  alphaK1 : Math  SaturateOnIntegerOverflow=on
  betaK : Math  SaturateOnIntegerOverflow=on
  betaK1 : Math  SaturateOnIntegerOverflow=on
  c : Constant  Value=23
  c1 : Constant  Value=12
  c10 : Gain  Gain=1/10
  c{5,8..9,11..12,17,20,23,29} (9 alike) : Constant
  c13 : Gain  Gain=-0.2
  c14 : Constant  Value=29
  c15 : Gain  Gain=1/10
  c16 : Gain  Gain=0.23
  c18 : Constant  Value=3
  c19 : Constant  Value=1000
  c2 : Gain  Gain=1/46
  c21 : Constant  Value=-1/1000
  c22 : Constant  Value=1/2
  c24 : Constant  Value=-2
  c25 : Constant  Value=1000000
  c26 : Constant  Value=1/1000
  c27 : Constant  Value=-2
  c28 : Constant  Value=1/1000
  c3 : Gain  Gain=0.6
  c30 : Constant  Value=1000
  c31 : Constant  Value=1000
  c32 : Gain  Gain=0.00001
  c33 : Gain  Gain=0.1
  c34 : Gain  Gain=0.01
  c4 : Gain  Gain=1/23
  c6 : Constant  Value=12
  c7 : Gain  Gain=0.01
  "gg " : Gain  Gain=1000
  gk : Constant  Value=9.6
  kb : Gain  Gain=-0.3
  kb1 : Gain  Gain=0.3
  kf : Gain  Gain=0.1
  kf1 : Gain  Gain=-0.1
  mCa : Math  Operator=square  SaturateOnIntegerOverflow=on
  mk : Math  Operator=pow  SaturateOnIntegerOverflow=on
  V : Outport
  "Cain " : Outport  Port=2
  ICa : Outport  Port=3
  IK : Outport  Port=4
  Isk : Outport  Port=5
  Ileak : Outport  Port=6
  wires:
  Divide/1 -> Product1/2  "BetaK"
  c10/1 -> betaK1/1
  Sum7/1 -> Divide1/2
  c/1 -> Sum/2
  R/1 -> T/1
  c3/1 -> Product/1  "alphaK"
  c9/1 -> Sum6/2
  c6/1 -> Sum3/2
  Product/1 -> Sum5/1
  Sum1/1 -> c4/1
  c13/1 -> Divide1/1
  Caout1/1 -> Sum19/1
  T/1 -> Divide3/2
  Ksk/1 -> Sum20/2
  Product14/1 -> Ileak/1, Sum24/7  "Ileak"
  Sum24/1 -> "Cm "/1
  "Cm "/1 -> Integrator7/1  "dv/dt"
  Divide3/1 -> Caout/1
  c31/1 -> Product14/3
  Integrator6/1 -> Sum21/2, Product13/1  "msk"
  Sum21/1 -> Divide7/1
  Sum23/1 -> Product14/2
  Divide6/1 -> Sum21/1
  c12/1 -> Sum8/2
  Integrator3/1 -> Product3/1, mCa/1, Sum10/1  "mCa"
  Sum5/1 -> Integrator2/1  "dmk/dt"
  c15/1 -> alphaK1/1
  Sum9/1 -> c15/1
  c2/1 -> alphaK/1
  Sum22/1 -> Product13/3
  Product10/1 -> Divide5/1
  Integrator2/1 -> mk/1, Product1/1, Sum4/1  "mk"
  Divide8/1 -> Divide7/2
  R1/1 -> T1/1
  Caout/1 -> "Caout "/1
  Sum3/1 -> c7/1
  Sum6/1 -> c10/1
  Divide4/1 -> Caout1/1
  c30/1 -> Product13/4
  c28/1 -> Product12/3
  c11/1 -> Sum7/2
  betaK1/1 -> Sum7/1
  Divide7/1 -> Integrator6/1  "dmsk/dt"
  Ichem/1 -> Sum24/4
  c7/1 -> Divide/1
  Sum14/1 -> Product5/1
  Sum13/1 -> Integrator4/1  "dCaB/dt"
  Integrator5/1 -> Sum20/1, Divide6/1, Product9/1, Sum17/1, Product8/3, "Cain "/1, Sum18/2, Product5/2  "Cain"
  c21/1 -> Product6/1
  c22/1 -> Product6/2
  1/F/1 -> Product6/3
  1/d/1 -> Product6/4
  c25/1 -> Product6/5
  "gg "/1 -> Sum24/2, ICa/1, Product6/6  "ICa"
  B/1 -> Product8/1, kb1/1
  kb1/1 -> Product7/2
  Product7/1 -> Sum15/1
  Product5/1 -> kf/1
  kf/1 -> Sum13/2
  c23/1 -> Sum16/2
  Sum16/1 -> kf1/1
  kf1/1 -> Product8/2
  Product8/1 -> Sum15/2
  Product6/1 -> Sum15/3
  Product9/1 -> Divide2/1
  Kpump/1 -> Sum17/2
  Sum17/1 -> Divide2/2
  Divide2/1 -> Sum15/4
  Sum15/1 -> Integrator5/1  "dCain/dt"
  mCa/1 -> Product10/1  "mCa^2"
  c24/1 -> Product11/1
  F/1 -> Product11/2
  c26/1 -> Product11/3
  Integrator7/1 -> V/1, Sum22/2, Product11/4, Product10/3, Sum6/1, Sum1/1, Sum3/1, Sum/1, Sum12/1, Sum8/1, Sum9/1, Product12/4, Sum23/2  "v"
  c14/1 -> Sum9/2
  Saisk/1 -> Divide8/1
  Sum18/1 -> Product10/4
  Iinput/1 -> Sum24/3
  "Caout "/1 -> Sum18/1
  Sum/1 -> c2/1
  Sum8/1 -> c13/1
  c16/1 -> Product3/2  "BetaCa"
  Product11/1 -> Divide3/1
  T1/1 -> Divide4/2
  betaK/1 -> Sum2/1
  c29/1 -> Sum19/2
  Product1/1 -> Sum5/2
  c4/1 -> betaK/1
  alphaK/1 -> c3/1
  alphaK1/1 -> c16/1
  Divide1/1 -> Product2/1  "AlphaCa"
  Sum2/1 -> Divide/2
  Sum4/1 -> Product/2  "1-mk"
  c5/1 -> Sum2/2
  c8/1 -> Sum4/2
  Igap/1 -> Sum24/5
  Product13/1 -> Isk/1, Sum24/6  "Isk"
  Divide5/1 -> "gg "/1
  Sum20/1 -> Divide8/2, Divide6/2
  Product12/1 -> Divide4/1
  c27/1 -> Product12/1
  F1/1 -> Product12/2
  c1/1 -> Sum1/2
  Sum11/1 -> Integrator3/1  "dmCa/dt"
  c17/1 -> Sum10/2
  "Ek "/1 -> Sum26/1
  Sum10/1 -> Product2/2  "1-mCa"
  Sum12/1 -> Product4/3
  Product3/1 -> Sum11/2
  Product4/1 -> IK/1, Sum24/1  "IK"
  Integrator4/1 -> Product7/1, Sum16/1, Sum14/1, kb/1  "CaB"
  kb/1 -> Sum13/1
  c20/1 -> Sum14/2
  mk/1 -> Product4/2
  Random/1 -> c32/1, c33/1, Sum28/2, Sum30/2, Sum25/2, Sum26/2, Sum32/2, c34/1
  c19/1 -> Product4/4
  Product2/1 -> Sum11/1
  c18/1 -> mk/2
  Sum19/1 -> Divide5/2
  gk/1 -> Sum25/1
  Sum25/1 -> Product4/1
  Sum26/1 -> Sum12/2
  Pmax/1 -> Sum27/1
  Sum27/1 -> Product10/2
  Sum28/1 -> Product9/2
  Gpump/1 -> Sum28/1
  Sum29/1 -> Product13/2
  Gsk/1 -> Sum29/1
  Sum30/1 -> Sum22/1
  Esk/1 -> Sum30/1
  Gleak/1 -> Sum31/1
  Sum31/1 -> Product14/1
  Sum32/1 -> Sum23/1
  Eleak/1 -> Sum32/1
  c32/1 -> Sum27/2
  c33/1 -> Sum29/2
  c34/1 -> Sum31/2

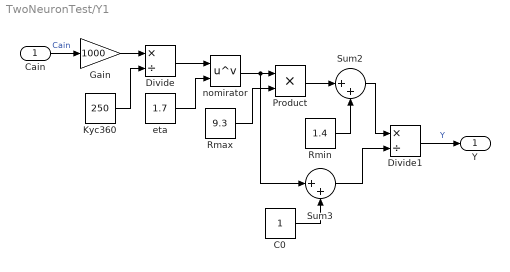
== system TwoNeuronTest/Y1 ==
  Cain : Inport
  C0 : Constant
  Divide : Product  Inputs=*/
  Divide1 : Product  Inputs=*/
  Gain : Gain  Gain=1000
  Kyc360 : Constant  Value=250
  Product : Product
  Rmax : Constant  Value=9.3
  Rmin : Constant  Value=1.4
  Sum2 : Sum  Inputs=|++
  Sum3 : Sum  Inputs=|++
  eta : Constant  Value=1.7
  nomirator : Math  Operator=pow  SaturateOnIntegerOverflow=on
  Y : Outport
  wires:
  nomirator/1 -> Sum3/1, Product/1
  Cain/1 -> Gain/1  "Cain"
  C0/1 -> Sum3/2
  Divide/1 -> nomirator/1
  eta/1 -> nomirator/2
  Rmin/1 -> Sum2/2
  Product/1 -> Sum2/1
  Sum2/1 -> Divide1/1
  Divide1/1 -> Y/1  "Y"
  Gain/1 -> Divide/1
  Rmax/1 -> Product/2
  Sum3/1 -> Divide1/2
  Kyc360/1 -> Divide/2

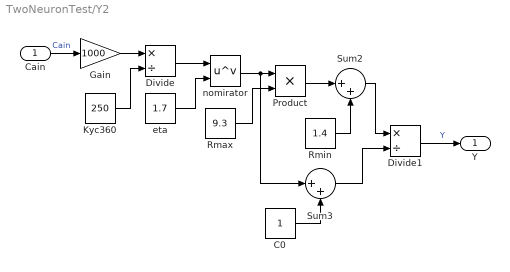
== system TwoNeuronTest/Y2 ==
  Cain : Inport
  C0 : Constant
  Divide : Product  Inputs=*/
  Divide1 : Product  Inputs=*/
  Gain : Gain  Gain=1000
  Kyc360 : Constant  Value=250
  Product : Product
  Rmax : Constant  Value=9.3
  Rmin : Constant  Value=1.4
  Sum2 : Sum  Inputs=|++
  Sum3 : Sum  Inputs=|++
  eta : Constant  Value=1.7
  nomirator : Math  Operator=pow  SaturateOnIntegerOverflow=on
  Y : Outport
  wires:
  nomirator/1 -> Sum3/1, Product/1
  Cain/1 -> Gain/1  "Cain"
  C0/1 -> Sum3/2
  Divide/1 -> nomirator/1
  eta/1 -> nomirator/2
  Rmin/1 -> Sum2/2
  Product/1 -> Sum2/1
  Sum2/1 -> Divide1/1
  Divide1/1 -> Y/1  "Y"
  Gain/1 -> Divide/1
  Rmax/1 -> Product/2
  Sum3/1 -> Divide1/2
  Kyc360/1 -> Divide/2
